simulink model "saturation_nonlinearity"  (R2024a)
settings: Solver=FixedStepAuto  StartTime=0.0  StopTime=35  FixedStep=1e-6  RelTol=1e-3
settings Model: Creator=Lenovo  LastModifiedBy=Lenovo

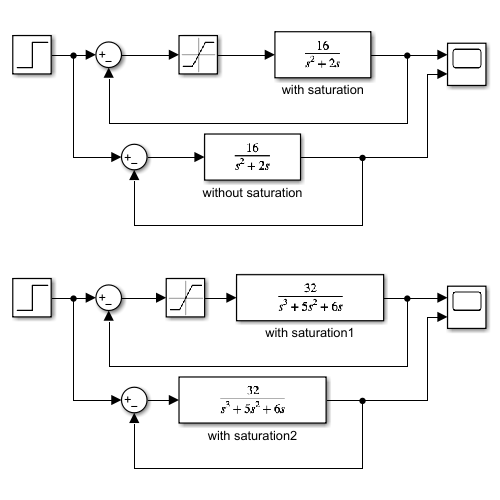
[thumbnail: Simulink's stored preview of the top-level diagram]
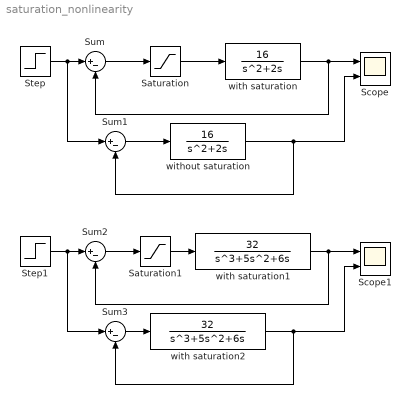
== system saturation_nonlinearity ==
  Saturation : Saturate
  Saturation1 : Saturate
  Scope : Scope  NumInputPorts=2
  Scope1 : Scope  NumInputPorts=2
  Step : Step  SampleTime=0
  Step1 : Step  SampleTime=0
  Sum{,1..3} (4 alike) : Sum  Inputs=|+-
  with saturation : TransferFcn  Numerator=[16]  Denominator=[1 2 0]
  with saturation1 : TransferFcn  Numerator=[32]  Denominator=[1,5,6,0]
  with saturation2 : TransferFcn  Numerator=[32]  Denominator=[1,5,6,0]
  without saturation : TransferFcn  Numerator=[16]  Denominator=[1 2 0]
  wires:
  Sum/1 -> Saturation/1
  Saturation/1 -> with saturation/1
  with saturation/1 -> Scope/1, Sum/2
  without saturation/1 -> Scope/2, Sum1/2
  Step/1 -> Sum1/1, Sum/1
  Sum1/1 -> without saturation/1
  Step1/1 -> Sum2/1, Sum3/1
  with saturation2/1 -> Sum3/2, Scope1/2
  with saturation1/1 -> Sum2/2, Scope1/1
  Saturation1/1 -> with saturation1/1
  Sum2/1 -> Saturation1/1
  Sum3/1 -> with saturation2/1
